simulink subsystem "Intake_Rollers_and_Shooter_Wheels"  (R2023b)
settings: Solver=VariableStepAuto  StartTime=0.0  StopTime=10.0  RelTol=1e-3
undefined symbols (not defined in the file): Note_Detect_Dist_Intake, Note_Detect_Dist_Shooter, Note_Time_Eject, Note_Time_Speaker_Spin_Up, Note_Time_Transfer, Note_Time_Transfer_Spin_Up, Servo_Addition_out, Servo_Front_Arm_Length_in, Servo_Store_Gain, Servo_Store_Offset, Servo_Time_Deploy, Servo_Time_Store, Shooter_DC_Eject, Shooter_Motor_DesSpd_Store, Shooter_Motor_Speed_Transition, t_sample, TEST_Servo_Override_Flag, TEST_Servo_Override_Value
libraries: simulink x13, Controls_Components_lib x2
settings Model: Creator=ander  LastModifiedBy=FIRSTMentor

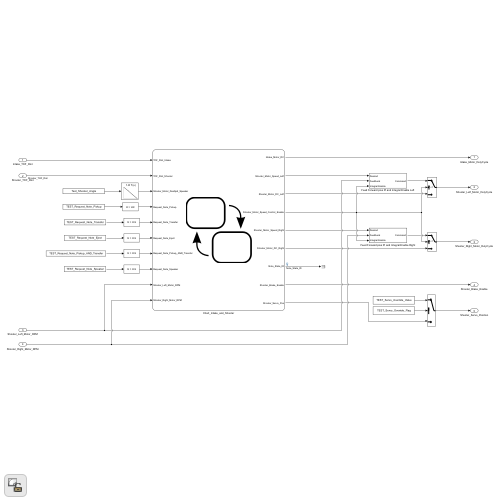
[thumbnail: Simulink's stored preview of the top-level diagram]
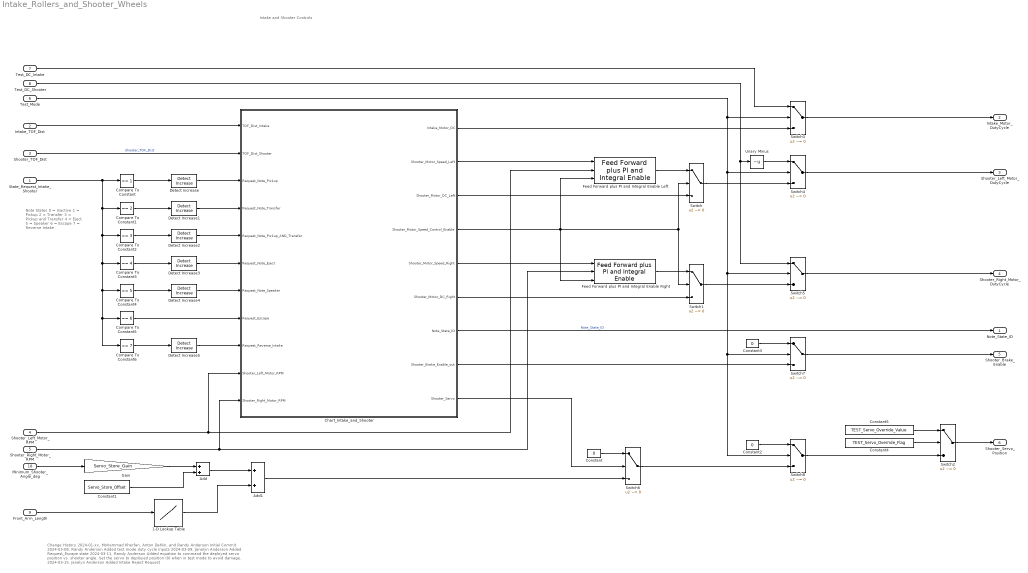
== system Intake_Rollers_and_Shooter_Wheels ==
  note: Intake and Shooter Controls
  note: Change History
      | 2024-01-xx, Mohammad Kherfan, Anton Dahlin, and Randy Anderson
      | Initial Commit
      | 2024-03-08, Randy Anderson
      | Added test mode duty cycle inputs
      | 2024-03-09, Janelyn Anderson
      | Added Request_Escape state
      | 2024-03-11, Randy Anderson
      | Added equation to command the deployed servo position vs. shooter angle.
      | Set the servo to deployed position (0) when in test mode to avoid damage.
      | 2024-03-15, Janelyn Anderson
      | Added Intake Reject Request
  note: Note States
      | 0 = Inactive
      | 1 = Pickup
      | 2 = Transfer
      | 3 = Pickup and Transfer
      | 4 = Eject
      | 5 = Speaker
      | 6 = Escape
      | 7 = Reverse Intake
  State_Request_Intake_Shooter : Inport
  Intake_TOF_Dist : Inport  Port=2
  Shooter_TOF_Dist : Inport  Port=3
  Shooter_Left_Motor_RPM : Inport  Port=4
  Shooter_Right_Motor_RPM : Inport  Port=5
  Test_Mode : Inport  Port=6
  Test_DC_Intake : Inport  Port=7
  Test_DC_Shooter : Inport  Port=8
  Front_Arm_Length : Inport  Port=9
  Minimum_Shooter_Angle_deg : Inport  Port=10
  1-D Lookup Table : Lookup_n-D  NumberOfTableDimensions=1  BreakpointsForDimension1=Servo_Front_Arm_Length_in  Table=Servo_Addition_out  ExtrapMethod=Clip  InternalRulePriority=Speed  RndMeth=Simplest
  Add : Sum
  Add1 : Sum
  Chart_Intake_and_Shooter : Stateflow chart  TreatAsAtomicUnit=on
      settings: PortSchema="{\"entries\":[{\"content\":{\"sides\":[{\"content\":{\"connectorIds\":[\"In1\",\"In2\",\"In3\",\"In4\",\"In6\",\"In5\",\"In7\",\"In8\",\"In11\",\"In9\",\"In10\"]},\"type\":\"ConnectorPlacement.EquallySpacedRectSide\",\"uuid\":\"d4f7d716-e95d-470b-97b3-4201307aef8b\"},{\"content\":{\"connectorIds\":[\"Out1\",\"Out2\",\"Out3\",\"Out4\",\"Out5\",\"Out6\",\"Out7\",\"Out8\",\"Out9\"],\"side\":\"RIGHT\"},\"type\":\"ConnectorPlacement.EquallySpacedRectSide\",\"uuid\":\"0a4b3d24-6288-4c9f-b07a-353227d48820\"},{\"content\":{\"side\":\"TOP\"},\"type\":\"ConnectorPlacement.EquallySpacedRectSide\",\"uuid\":\"1a2e556d-c5a0-4ed4-bdc8-45ca536baade\"}]},\"type\":\"ConnectorPlacement.EquallySpacedConnector\",\"uuid\":\"a3deefcc-177a-4af9-b921-4ee532472f51\"}],\"packageUris\":[\"http://schema.mathworks.com/mf0/Connector/R2020b\"],\"version\":\"1.0\"}"
  Compare To Constant : simulink/Logic and Bit Operations/Compare To Constant  relop===  const=1  OutDataTypeStr=boolean
  Compare To Constant1 : simulink/Logic and Bit Operations/Compare To Constant  relop===  const=2  OutDataTypeStr=boolean
  Compare To Constant2 : simulink/Logic and Bit Operations/Compare To Constant  relop===  const=3  OutDataTypeStr=boolean
  Compare To Constant3 : simulink/Logic and Bit Operations/Compare To Constant  relop===  const=4  OutDataTypeStr=boolean
  Compare To Constant4 : simulink/Logic and Bit Operations/Compare To Constant  relop===  const=5  OutDataTypeStr=boolean
  Compare To Constant5 : simulink/Logic and Bit Operations/Compare To Constant  relop===  const=6  OutDataTypeStr=boolean
  Compare To Constant6 : simulink/Logic and Bit Operations/Compare To Constant  relop===  const=7  OutDataTypeStr=boolean
  Constant : Constant  Value=0
  Constant1 : Constant  Value=Servo_Store_Offset
  Constant2 : Constant  Value=0
  Constant3 : Constant  Value=0
  Constant4 : Constant  Value=TEST_Servo_Override_Flag
  Constant5 : Constant  Value=TEST_Servo_Override_Value
  Detect Increase{,1..5} (6 alike) : simulink/Logic and Bit Operations/Detect Increase  vinit=0.0  OutDataTypeStr=boolean
  Feed Forward plus PI and Integral Enable Left : Controls_Components_lib/Feed Forward plus PI and Integral Enable  Gain_FF=Shooter_Motor_Control_FF  Gain_P=Shooter_Motor_Control_P  Gain_I=Shooter_Motor_Control_I  Limit_I_Upper=Shooter_Motor_Control_I_UL  Limit_I_Lower=Shooter_Motor_Control_I_LL  Limit_T_Upper=1  Limit_T_Lower=-1
  Feed Forward plus PI and Integral Enable Right : Controls_Components_lib/Feed Forward plus PI and Integral Enable  Gain_FF=Shooter_Motor_Control_FF  Gain_P=Shooter_Motor_Control_P  Gain_I=Shooter_Motor_Control_I  Limit_I_Upper=Shooter_Motor_Control_I_UL  Limit_I_Lower=Shooter_Motor_Control_I_LL  Limit_T_Upper=1  Limit_T_Lower=-1
  Gain : Gain  Gain=Servo_Store_Gain
  Switch{,1..8} (9 alike) : Switch  Criteria=u2 ~= 0  SaturateOnIntegerOverflow=off  InputSameDT=off
  Unary Minus : UnaryMinus
  Note_State_ID : Outport
  Intake_Motor_DutyCycle : Outport  Port=2
  Shooter_Left_Motor_DutyCycle : Outport  Port=3
  Shooter_Right_Motor_DutyCycle : Outport  Port=4
  Shooter_Brake_Enable : Outport  Port=5
  Shooter_Servo_Position : Outport  Port=6
  wires:
  Intake_TOF_Dist/1 -> Chart_Intake_and_Shooter/1(TOF_Dist_Intake)
  Chart_Intake_and_Shooter/1(Intake_Motor_DC) -> Switch3/3
  Shooter_TOF_Dist/1 -> Chart_Intake_and_Shooter/2(TOF_Dist_Shooter)  "Shooter_TOF_Dist"
  Chart_Intake_and_Shooter/7(Note_State_ID) -> Note_State_ID/1  "Note_State_ID"
  Chart_Intake_and_Shooter/2(Shooter_Motor_Speed_Left) -> Feed Forward plus PI and Integral Enable Left/1
  Shooter_Left_Motor_RPM/1 -> Feed Forward plus PI and Integral Enable Left/2, Chart_Intake_and_Shooter/9(Shooter_Left_Motor_RPM)
  Chart_Intake_and_Shooter/5(Shooter_Motor_Speed_Right) -> Feed Forward plus PI and Integral Enable Right/1
  Shooter_Right_Motor_RPM/1 -> Feed Forward plus PI and Integral Enable Right/2, Chart_Intake_and_Shooter/10(Shooter_Right_Motor_RPM)
  Chart_Intake_and_Shooter/3(Shooter_Motor_DC_Left) -> Switch/3
  Chart_Intake_and_Shooter/6(Shooter_Motor_DC_Right) -> Switch1/3
  Chart_Intake_and_Shooter/4(Shooter_Motor_Speed_Control_Enable) -> Feed Forward plus PI and Integral Enable Right/3, Switch1/2, Switch/2, Feed Forward plus PI and Integral Enable Left/3
  Feed Forward plus PI and Integral Enable Left/1 -> Switch/1
  Feed Forward plus PI and Integral Enable Right/1 -> Switch1/1
  Detect Increase/1 -> Chart_Intake_and_Shooter/3(Request_Note_Pickup)
  Detect Increase1/1 -> Chart_Intake_and_Shooter/4(Request_Note_Transfer)
  Switch2/1 -> Shooter_Servo_Position/1
  Detect Increase4/1 -> Chart_Intake_and_Shooter/7(Request_Note_Speaker)
  State_Request_Intake_Shooter/1 -> Compare To Constant1/1, Compare To Constant2/1, Compare To Constant3/1, Compare To Constant4/1, Compare To Constant5/1, Compare To Constant6/1, Compare To Constant/1
  Compare To Constant1/1 -> Detect Increase1/1
  Compare To Constant2/1 -> Detect Increase2/1
  Compare To Constant3/1 -> Detect Increase3/1
  Compare To Constant4/1 -> Detect Increase4/1
  Detect Increase2/1 -> Chart_Intake_and_Shooter/6(Request_Note_Pickup_AND_Transfer)
  Detect Increase3/1 -> Chart_Intake_and_Shooter/5(Request_Note_Eject)
  Switch3/1 -> Intake_Motor_DutyCycle/1
  Switch/1 -> Switch4/3
  Switch1/1 -> Switch5/3
  Switch5/1 -> Shooter_Right_Motor_DutyCycle/1
  Switch4/1 -> Shooter_Left_Motor_DutyCycle/1
  Test_Mode/1 -> Switch3/2, Switch4/2, Switch5/2, Switch8/2, Switch7/2
  Test_DC_Intake/1 -> Switch3/1
  Test_DC_Shooter/1 -> Unary Minus/1, Switch5/1
  Unary Minus/1 -> Switch4/1
  Compare To Constant5/1 -> Chart_Intake_and_Shooter/8(Request_Escape)
  Constant4/1 -> Switch2/2
  Constant5/1 -> Switch2/1
  Chart_Intake_and_Shooter/9(Shooter_Servo) -> Switch6/2
  Constant/1 -> Switch6/1
  Minimum_Shooter_Angle_deg/1 -> Gain/1
  Gain/1 -> Add/1
  Constant1/1 -> Add/2
  Add1/1 -> Switch6/3
  Switch8/1 -> Switch2/3
  Switch6/1 -> Switch8/3
  Constant2/1 -> Switch8/1
  Compare To Constant/1 -> Detect Increase/1
  Switch7/1 -> Shooter_Brake_Enable/1
  Chart_Intake_and_Shooter/8(Shooter_Brake_Enable_out) -> Switch7/3
  Constant3/1 -> Switch7/1
  Front_Arm_Length/1 -> 1-D Lookup Table/1
  Add/1 -> Add1/1
  1-D Lookup Table/1 -> Add1/2
  Compare To Constant6/1 -> Detect Increase5/1
  Detect Increase5/1 -> Chart_Intake_and_Shooter/11(Request_Reverse_Intake)

== stateflow chart Intake_Rollers_and_Shooter_Wheels/Chart_Intake_and_Shooter ==
  state Note_Speaker_Score_Intake
    en: Note_State_ID = 5.3;
    Intake_Motor_DC = -1;
  state Note_Intake_AND_Shooter
    en: Note_State_ID = 4.1;
    Intake_Motor_DC = -1;
    Shooter_Servo = Servo_Up;
    Shooter_Brake_Enable_out = 0;
    Shooter_Motor_Speed_Control_Enable = 1;
    Shooter_Motor_Speed_Left = -Shooter_Motor_DesSpd_Store;
    Shooter_Motor_Speed_Right = Shooter_Motor_DesSpd_Store;
  state Extra_Run_Time6
    en: Note_State_ID = 5.2;
    timer = t_sample;
    du: timer = timer + t_sample;
  note: There isn't a state here waiting for the Servo to deploy because it is assumed that it will take at least that amount of time to get the note through the intake.
  state Note_Speaker_Score_SpinUp
    en: Note_State_ID = 5.1;
    Shooter_Servo = Servo_Down;
    Shooter_Brake_Enable_out = 0;
    Shooter_Motor_Speed_Control_Enable = 0;
    Shooter_Motor_DC_Left = -1;
    Shooter_Motor_DC_Right = 1;
    //Shooter_Motor_Speed_Left = -Shooter_Motor_DesSpd_Speaker;
    //Shooter_Motor_Speed_Right = Shooter_Motor_DesSpd_Speaker;
    //du: Shooter_Motor_Speed_Left = -Shooter_Motor_DesSpd_Speaker;
    // Shooter_Motor_Speed_Right = Shooter_Motor_DesSpd_Speaker;
  state Extra_Run_Time4
    en: Note_State_ID = 4.2;
    timer = t_sample;
    du: timer = timer + t_sample;
  state Extra_Run_Time5
    en: Note_State_ID = 5.4;
    timer = t_sample;
    du: timer = timer + t_sample;
  state Store_Servo
    en: Note_State_ID = 3.1;
    Shooter_Servo = Servo_Down;
    timer = t_sample;
    du: timer = timer + t_sample;
  state Note_Eject_from_Shooter
    en: Note_State_ID = 3.2;
    Shooter_Brake_Enable_out = 0;
    Shooter_Motor_DC_Left = -Shooter_DC_Eject;
    Shooter_Motor_DC_Right = Shooter_DC_Eject;
    timer = t_sample;
    du: timer = timer + t_sample;
  state Waiting_for_Requests
    en: Note_State_ID = 0;
    Intake_Motor_DC = 0;
    Shooter_Brake_Enable_out = 1;
    Shooter_Motor_Speed_Control_Enable = 0;
    Shooter_Motor_DC_Left = 0;
    Shooter_Motor_DC_Right = 0;
  state Note_Pickup
    en: Note_State_ID = 1;
    Intake_Motor_DC = -1;
    Shooter_Servo = Servo_Down;
  state Spin_Up_Shooter_Before_Transfer
    en: Note_State_ID = 2.1;
    Shooter_Servo = Servo_Up;
    Shooter_Brake_Enable_out = 0;
    Shooter_Motor_Speed_Control_Enable = 1;
    Shooter_Motor_Speed_Left = -Shooter_Motor_DesSpd_Store;
    Shooter_Motor_Speed_Right = Shooter_Motor_DesSpd_Store;
    timer = t_sample;
    du: timer = timer + t_sample;
  state Reverse_Intake
    en: Note_State_ID = 6.1;
    Intake_Motor_DC = 1;
    timer = t_sample;
    du:
    timer = timer + t_sample;
  state Extra_Run_Time2
    en: Note_State_ID = 2.3;
    timer = t_sample;
    du: timer = timer + t_sample;
  state Note_Transfer_to_Shooter
    en: Note_State_ID = 2.2;
    Intake_Motor_DC = -1;
  Note_Speaker_Score_Intake -> Extra_Run_Time5 : [TOF_Dist_Intake > Note_Detect_Dist_Intake ||...
      | Request_Escape]
  Extra_Run_Time6 -> Note_Speaker_Score_Intake [order 1] : [timer >= Note_Time_Speaker_Spin_Up]
  Extra_Run_Time6 -> Note_Speaker_Score_SpinUp [order 2] : [Request_Escape]
  Note_Speaker_Score_SpinUp -> Extra_Run_Time6 [order 1] : [Shooter_Left_Motor_RPM < -Shooter_Motor_Speed_Transition && ...
      | Shooter_Right_Motor_RPM > Shooter_Motor_Speed_Transition]
  Note_Intake_AND_Shooter -> Extra_Run_Time4 : [TOF_Dist_Shooter <= Note_Detect_Dist_Shooter ||...
      | Request_Escape]
  Waiting_for_Requests -> Note_Intake_AND_Shooter [order 1] : [Request_Note_Pickup_AND_Transfer]
  Extra_Run_Time4 -> Waiting_for_Requests : [timer >= Note_Time_Transfer ||...
      | Request_Escape]
  Extra_Run_Time5 -> Waiting_for_Requests : [timer >= Note_Time_Eject ||...
      | Request_Escape]
  Note_Speaker_Score_SpinUp -> Waiting_for_Requests [order 2] : [Request_Escape]
  Waiting_for_Requests -> Note_Speaker_Score_SpinUp [order 5] : [Request_Note_Speaker]
  (default) -> Waiting_for_Requests : {Shooter_Servo = Servo_Down;}
  Waiting_for_Requests -> Store_Servo [order 4] : [Request_Note_Eject]
  Store_Servo -> Note_Eject_from_Shooter [order 1] : [timer >= Servo_Time_Store]
  Waiting_for_Requests -> Note_Pickup [order 3] : [Request_Note_Pickup]
  Store_Servo -> Waiting_for_Requests [order 2] : [Request_Escape]
  Note_Pickup -> Waiting_for_Requests : [TOF_Dist_Intake <= Note_Detect_Dist_Intake ||...
      | Request_Escape]
  Note_Eject_from_Shooter -> Waiting_for_Requests : [timer >= Note_Time_Eject ||...
      | Request_Escape]
  Extra_Run_Time2 -> Waiting_for_Requests [order 1] : [Request_Escape]
      | {Shooter_Servo = Servo_Down;}
  Extra_Run_Time2 -> Waiting_for_Requests [order 2] : [timer >= Note_Time_Transfer]
  Spin_Up_Shooter_Before_Transfer -> Waiting_for_Requests [order 2] : [Request_Escape]
      | {Shooter_Servo = Servo_Down;}
  Waiting_for_Requests -> Spin_Up_Shooter_Before_Transfer [order 2] : [Request_Note_Transfer]
  Waiting_for_Requests -> Reverse_Intake [order 6] : [Request_Reverse_Intake]
  Reverse_Intake -> Waiting_for_Requests : [timer > 5 || Request_Escape]
  Note_Transfer_to_Shooter -> Extra_Run_Time2 : [TOF_Dist_Shooter <= Note_Detect_Dist_Shooter || ...
      | Request_Escape]
  Spin_Up_Shooter_Before_Transfer -> Note_Transfer_to_Shooter [order 1] : [timer >= Note_Time_Transfer_Spin_Up && ...
      | timer >= Servo_Time_Deploy]
  data: TOF_Dist_Intake input double size=1; TOF_Dist_Shooter input double size=1; Intake_Motor_DC output double size=1; Shooter_Motor_Speed_Left output double size=1; Request_Note_Pickup input boolean size=1; Note_Detect_Dist_Intake parameter double size=1; Request_Note_Transfer input boolean size=1; t_sample parameter double size=1; timer local double size=1; Shooter_Motor_DC_Left output double size=1; Shooter_Motor_Speed_Control_Enable output boolean size=1; Shooter_Motor_Speed_Right output double size=1; Shooter_Motor_DC_Right output double size=1; Request_Note_Eject input boolean size=1; Shooter_DC_Eject parameter double size=1; Note_Time_Eject parameter double size=1; Note_Detect_Dist_Shooter parameter double size=1; Note_State_ID output double size=1; Shooter_Motor_DesSpd_Store parameter double size=1; Note_Time_Transfer parameter double size=1; Note_Time_Transfer_Spin_Up parameter double size=1; Shooter_Brake_Enable_out output boolean size=1; Request_Note_Pickup_AND_Transfer input boolean size=1; Request_Note_Speaker input boolean size=1; Request_Escape input; Shooter_Servo output boolean size=1; Servo_Down constant boolean size=1 =0; Servo_Up constant boolean size=1 =1; Servo_Time_Store parameter double size=1; Servo_Time_Deploy parameter double size=1; Shooter_Left_Motor_RPM input double size=1; Shooter_Right_Motor_RPM input double size=1; Shooter_Motor_Speed_Transition parameter double size=1; Note_Time_Speaker_Spin_Up parameter double size=1; Request_Reverse_Intake input
